simulink model "A2"  (R2018b)
settings: Solver=VariableStepAuto  StartTime=0.0  StopTime=10  RelTol=1e-3
values from neighbouring files (symbols this model uses):
  A1 = [0 0 1 0 ; 0 0 0 1 ; 0 A132 A133 A134 ; 0 A142 A143 A144]    [NXTway_model.m]
  B1 = [0 0 ; 0 0 ; B13 B13 ; B14 B14]    [NXTway_model.m]
settings Model: Creator=jimve  LastModifiedBy=jimve

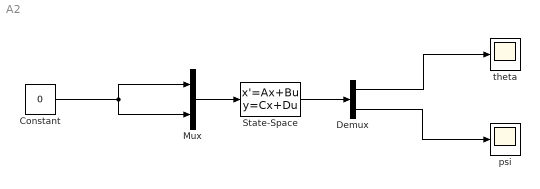
== system A2 ==
  Constant : Constant  Value=0
  Demux : Demux  Outputs=2
  Mux : Mux  Inputs=2
  State-Space : StateSpace  A=A1  B=B1  C=[1 0 0 0 ; 0 1 0 0]  D=zeros(2,2)  InitialCondition=[0 20 0 0]
  psi : Scope
  theta : Scope
  wires:
  State-Space/1 -> Demux/1
  Demux/1 -> theta/1
  Demux/2 -> psi/1
  Mux/1 -> State-Space/1
  Constant/1 -> Mux/2, Mux/1
